simulink model "REV3"  (R2025b)
settings: Solver=ode8  StartTime=0.0  StopTime=inf  FixedStep=0.0001  RelTol=1e-3
undefined symbols (not defined in the file): BMS_Contactor_Command, MC_DC_State, MC_VSM_State, UC_State
(part 1 of 2)
settings Model: DataDictionary=rev3_data.sldd  PacingRate=0.001000  Creator=rebek  LastModifiedBy=diego
settings DebuggingCC: ParameterPrecisionLossMsg=none
settings RTWCC: GPUComputeCapability=3.5

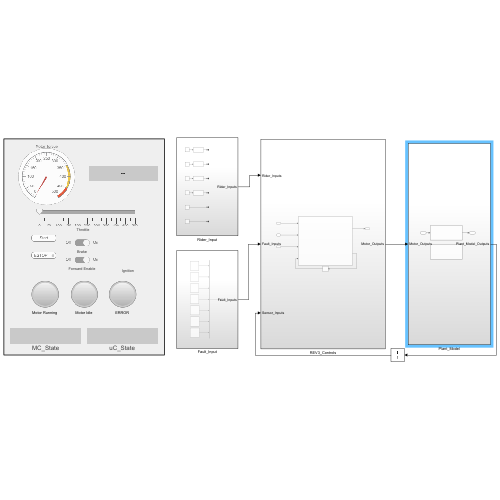
[thumbnail: Simulink's stored preview of the top-level diagram]
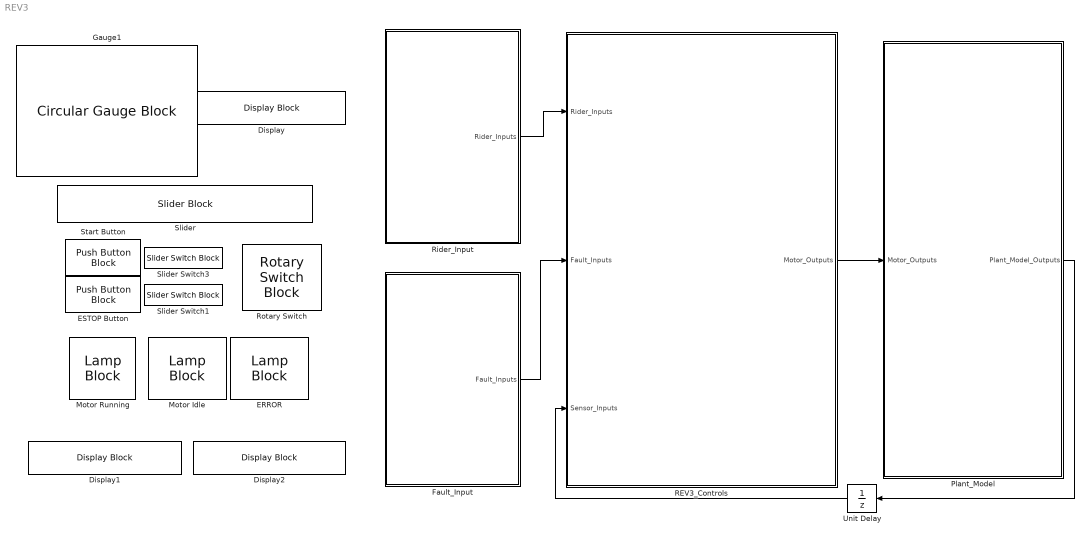
== system REV3 ==
  Display : DisplayBlock  LabelPosition=Hide  Transparency=1  GridColor=[0.502, 0.502, 0.502]
  Display1 : DisplayBlock  LabelPosition=Hide  Transparency=1  GridColor=[0.502, 0.502, 0.502]
      settings: AttributesFormatString=MC_State
  Display2 : DisplayBlock  LabelPosition=Hide  Transparency=1  GridColor=[0.502, 0.502, 0.502]
      settings: AttributesFormatString=uC_State
  ERROR : LampBlock  LabelPosition=Hide  DefaultColor=[192.0, 192.0, 192.0]
  ESTOP Button : PushButtonBlock  ButtonText=ESTOP  ButtonType=Latch  Icon=Circle  IconAlignment=Right  IconOnColor=[0.91764705882352937, 0.19607843137254902, 0.0392156862745098]  IconOffColor=[0.74901960784313726, 0.74901960784313726, 0.74901960784313726]  IconColor=On  OffValue=0.000000
  Fault_Input : Subsystem
  Gauge1 : CircularGaugeBlock  ScaleMax=500  FontColor=[0.0, 0.0, 0.0]
  Motor Idle : LampBlock  LabelPosition=Hide  DefaultColor=[192.0, 192.0, 192.0]
  Motor Running : LampBlock  LabelPosition=Hide  DefaultColor=[192.0, 192.0, 192.0]
  Plant_Model : Subsystem
  REV3_Controls : Subsystem
  Rider_Input : Subsystem
  Rotary Switch : RotarySwitchBlock  LabelPosition=Hide
      settings: AttributesFormatString=Ignition
  Slider : SliderBlock  LabelPosition=Hide  ScaleMax=500
      settings: AttributesFormatString=Throttle
  Slider Switch1 : SliderSwitchBlock  LabelPosition=Hide
      settings: AttributesFormatString=Forward Enable
  Slider Switch3 : SliderSwitchBlock  LabelPosition=Hide
      settings: AttributesFormatString=Brake
  Start Button : PushButtonBlock  ButtonText=Start  IconOnColor=[0.0, 0.39215686274509803, 0.0]  IconOffColor=[0.0, 1.0, 0.0]  OffValue=0.000000
  Unit Delay : UnitDelay  SampleTime=-1  HasFrameUpgradeWarning=on
  wires:
  Rider_Input/1(Rider_Inputs) -> REV3_Controls/1(Rider_Inputs)
  Fault_Input/1(Fault_Inputs) -> REV3_Controls/2(Fault_Inputs)
  REV3_Controls/1(Motor_Outputs) -> Plant_Model/1(Motor_Outputs)
  Plant_Model/1(Plant_Model_Outputs) -> Unit Delay/1
  Unit Delay/1 -> REV3_Controls/3(Sensor_Inputs)

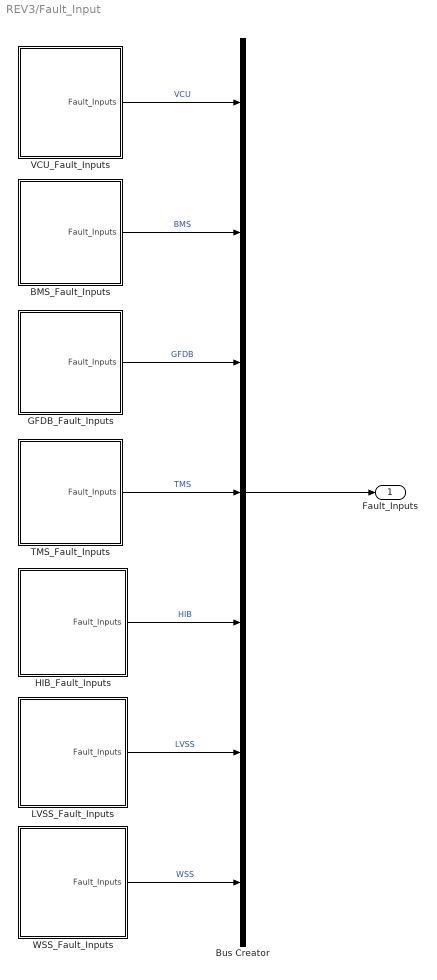
== system REV3/Fault_Input ==
  BMS_Fault_Inputs : Subsystem
  Bus Creator : BusCreator  Inputs=7
  GFDB_Fault_Inputs : Subsystem
  HIB_Fault_Inputs : Subsystem
  LVSS_Fault_Inputs : Subsystem
  TMS_Fault_Inputs : Subsystem
  VCU_Fault_Inputs : Subsystem
  WSS_Fault_Inputs : Subsystem
  Fault_Inputs : Outport
  wires:
  VCU_Fault_Inputs/1(Fault_Inputs) -> Bus Creator/1  "VCU"
  BMS_Fault_Inputs/1(Fault_Inputs) -> Bus Creator/2  "BMS"
  GFDB_Fault_Inputs/1(Fault_Inputs) -> Bus Creator/3  "GFDB"
  Bus Creator/1 -> Fault_Inputs/1
  TMS_Fault_Inputs/1(Fault_Inputs) -> Bus Creator/4  "TMS"
  HIB_Fault_Inputs/1(Fault_Inputs) -> Bus Creator/5  "HIB"
  LVSS_Fault_Inputs/1(Fault_Inputs) -> Bus Creator/6  "LVSS"
  WSS_Fault_Inputs/1(Fault_Inputs) -> Bus Creator/7  "WSS"

== system REV3/Plant_Model ==
  Motor_Outputs : Inport
  Bike_Orientation : Subsystem
  Wheel_Speed : Subsystem
  Plant_Model_Outputs : Outport
  wires:
  Motor_Outputs/1 -> Wheel_Speed/1(Motor_Outputs)
  Wheel_Speed/1(Plant_Model_Outputs) -> Plant_Model_Outputs/1

== system REV3/REV3_Controls ==
  Rider_Inputs : Inport
  Fault_Inputs : Inport  Port=2
  Sensor_Inputs : Inport  Port=3
  Control_Step : Subsystem
  Unit Delay : UnitDelay  SampleTime=-1  HasFrameUpgradeWarning=on
  Motor_Outputs : Outport
  wires:
  Rider_Inputs/1 -> Control_Step/1(Rider_Inputs)
  Fault_Inputs/1 -> Control_Step/2(Fault_Inputs)
  Unit Delay/1 -> Control_Step/4(Feedback_Input)
  Control_Step/1(Motor_Outputs) -> Motor_Outputs/1
  Control_Step/2(Feedback_Output) -> Unit Delay/1
  Sensor_Inputs/1 -> Control_Step/3(Sensor_Inputs)

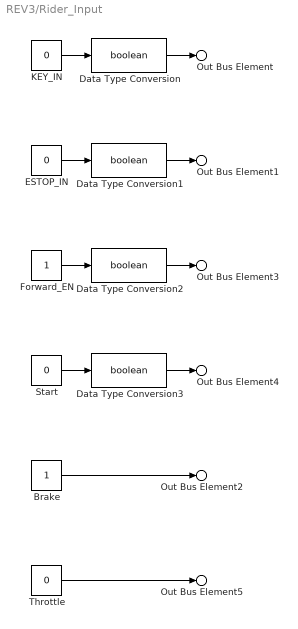
== system REV3/Rider_Input ==
  Brake : Constant
  Data Type Conversion{,1..3} (4 alike) : DataTypeConversion  OutDataTypeStr=boolean  SaturateOnIntegerOverflow=off  RndMeth=Floor
  ESTOP_IN : Constant  Value=0
  Forward_EN : Constant
  KEY_IN : Constant  Value=0
  Start : Constant  Value=0
  Throttle : Constant  Value=0  OutDataTypeStr=int16
  Out Bus Element5 : Outport  PortName=Rider_Inputs  Element=Yes_HIB.Throttle
  Out Bus Element4 : Outport  PortName=Rider_Inputs  Element=Yes_HIB.Start
  Out Bus Element3 : Outport  PortName=Rider_Inputs  Element=Yes_HIB.Forward_EN
  Out Bus Element2 : Outport  PortName=Rider_Inputs  Element=Yes_HIB.Brake
  Out Bus Element : Outport  PortName=Rider_Inputs  Element=No_HIB.Key_In
  Out Bus Element1 : Outport  PortName=Rider_Inputs  Element=No_HIB.Estop_In
  wires:
  KEY_IN/1 -> Data Type Conversion/1
  Brake/1 -> Out Bus Element2/1
  Data Type Conversion2/1 -> Out Bus Element3/1
  Data Type Conversion/1 -> Out Bus Element/1
  Forward_EN/1 -> Data Type Conversion2/1
  Data Type Conversion3/1 -> Out Bus Element4/1
  ESTOP_IN/1 -> Data Type Conversion1/1
  Throttle/1 -> Out Bus Element5/1
  Data Type Conversion1/1 -> Out Bus Element1/1
  Start/1 -> Data Type Conversion3/1

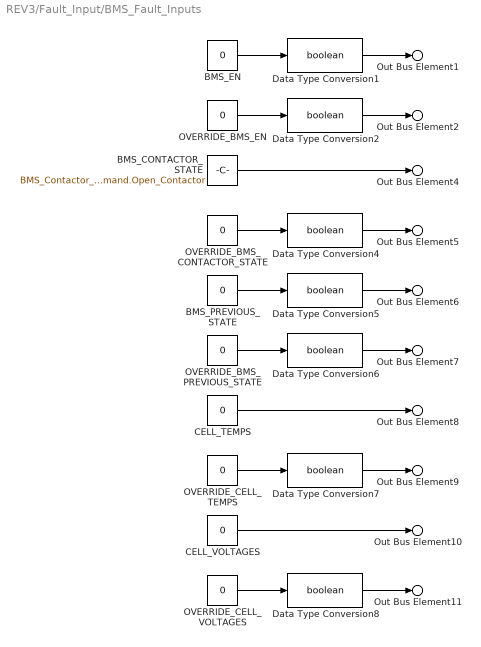
== system REV3/Fault_Input/BMS_Fault_Inputs ==
  BMS_CONTACTOR_STATE : Constant  Value=BMS_Contactor_Command.Open_Contactor  OutDataTypeStr=Enum: BMS_Contactor_Command
  BMS_EN : Constant  Value=0
  BMS_PREVIOUS_STATE : Constant  Value=0
  CELL_TEMPS : Constant  Value=0
  CELL_VOLTAGES : Constant  Value=0
  Data Type Conversion{1..2,4..8} (7 alike) : DataTypeConversion  OutDataTypeStr=boolean  SaturateOnIntegerOverflow=off  RndMeth=Floor
  OVERRIDE_BMS_CONTACTOR_STATE : Constant  Value=0
  OVERRIDE_BMS_EN : Constant  Value=0
  OVERRIDE_BMS_PREVIOUS_STATE : Constant  Value=0
  OVERRIDE_CELL_TEMPS : Constant  Value=0
  OVERRIDE_CELL_VOLTAGES : Constant  Value=0
  Out Bus Element4 : Outport  PortName=Fault_Inputs  Element=BMS_Contactor_State
  Out Bus Element5 : Outport  PortName=Fault_Inputs  Element=Override_BMS_Contactor_State
  Out Bus Element6 : Outport  PortName=Fault_Inputs  Element=BMS_Previous_State
  Out Bus Element7 : Outport  PortName=Fault_Inputs  Element=Override_BMS_Previous_State
  Out Bus Element8 : Outport  PortName=Fault_Inputs  Element=Cell_Temps
  Out Bus Element9 : Outport  PortName=Fault_Inputs  Element=Override_Cell_Temps
  Out Bus Element10 : Outport  PortName=Fault_Inputs  Element=Cell_Voltages
  Out Bus Element11 : Outport  PortName=Fault_Inputs  Element=Override_Cell_Voltages
  Out Bus Element1 : Outport  PortName=Fault_Inputs  Element=BMS_EN
  Out Bus Element2 : Outport  PortName=Fault_Inputs  Element=Override_BMS_EN
  wires:
  CELL_VOLTAGES/1 -> Out Bus Element10/1
  Data Type Conversion7/1 -> Out Bus Element9/1
  BMS_PREVIOUS_STATE/1 -> Data Type Conversion5/1
  OVERRIDE_CELL_TEMPS/1 -> Data Type Conversion7/1
  OVERRIDE_BMS_PREVIOUS_STATE/1 -> Data Type Conversion6/1
  BMS_CONTACTOR_STATE/1 -> Out Bus Element4/1
  OVERRIDE_CELL_VOLTAGES/1 -> Data Type Conversion8/1
  Data Type Conversion4/1 -> Out Bus Element5/1
  OVERRIDE_BMS_CONTACTOR_STATE/1 -> Data Type Conversion4/1
  Data Type Conversion5/1 -> Out Bus Element6/1
  Data Type Conversion6/1 -> Out Bus Element7/1
  CELL_TEMPS/1 -> Out Bus Element8/1
  Data Type Conversion8/1 -> Out Bus Element11/1
  Data Type Conversion2/1 -> Out Bus Element2/1
  Data Type Conversion1/1 -> Out Bus Element1/1
  BMS_EN/1 -> Data Type Conversion1/1
  OVERRIDE_BMS_EN/1 -> Data Type Conversion2/1

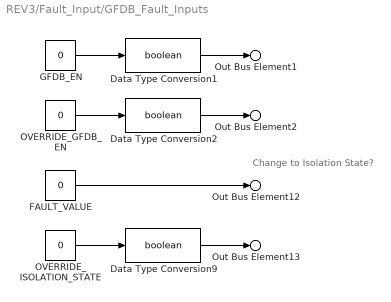
== system REV3/Fault_Input/GFDB_Fault_Inputs ==
  note: Change to Isolation State?
  Data Type Conversion1 : DataTypeConversion  OutDataTypeStr=boolean  SaturateOnIntegerOverflow=off  RndMeth=Floor
  Data Type Conversion2 : DataTypeConversion  OutDataTypeStr=boolean  SaturateOnIntegerOverflow=off  RndMeth=Floor
  Data Type Conversion9 : DataTypeConversion  OutDataTypeStr=boolean  SaturateOnIntegerOverflow=off  RndMeth=Floor
  FAULT_VALUE : Constant  Value=0
  GFDB_EN : Constant  Value=0
  OVERRIDE_GFDB_EN : Constant  Value=0
  OVERRIDE_ISOLATION_STATE : Constant  Value=0
  Out Bus Element12 : Outport  PortName=Fault_Inputs  Element=Fault_Value
  Out Bus Element13 : Outport  PortName=Fault_Inputs  Element=Override_Isolation_State
  Out Bus Element1 : Outport  PortName=Fault_Inputs  Element=GFDB_EN
  Out Bus Element2 : Outport  PortName=Fault_Inputs  Element=Override_GFDB_EN
  wires:
  FAULT_VALUE/1 -> Out Bus Element12/1
  Data Type Conversion9/1 -> Out Bus Element13/1
  OVERRIDE_ISOLATION_STATE/1 -> Data Type Conversion9/1
  OVERRIDE_GFDB_EN/1 -> Data Type Conversion2/1
  Data Type Conversion2/1 -> Out Bus Element2/1
  Data Type Conversion1/1 -> Out Bus Element1/1
  GFDB_EN/1 -> Data Type Conversion1/1

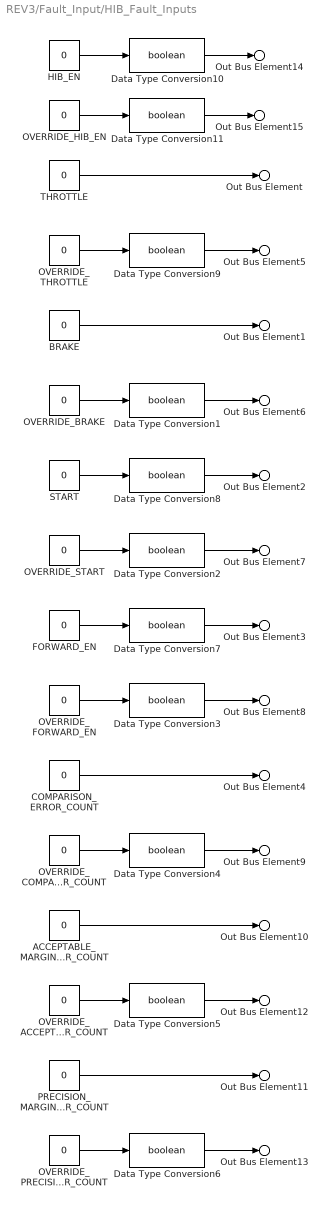
== system REV3/Fault_Input/HIB_Fault_Inputs ==
  ACCEPTABLE_MARGIN_ERROR_COUNT : Constant  Value=0
  BRAKE : Constant  Value=0
  COMPARISON_ERROR_COUNT : Constant  Value=0
  Data Type Conversion{1..11} (11 alike) : DataTypeConversion  OutDataTypeStr=boolean  SaturateOnIntegerOverflow=off  RndMeth=Floor
  FORWARD_EN : Constant  Value=0
  HIB_EN : Constant  Value=0
  OVERRIDE_ACCEPTABLE_MARGIN_ERROR_COUNT : Constant  Value=0
  OVERRIDE_BRAKE : Constant  Value=0
  OVERRIDE_COMPARISON_ERROR_COUNT : Constant  Value=0
  OVERRIDE_FORWARD_EN : Constant  Value=0
  OVERRIDE_HIB_EN : Constant  Value=0
  OVERRIDE_PRECISION_MARGIN_ERROR_COUNT : Constant  Value=0
  OVERRIDE_START : Constant  Value=0
  OVERRIDE_THROTTLE : Constant  Value=0
  PRECISION_MARGIN_ERROR_COUNT : Constant  Value=0
  START : Constant  Value=0
  THROTTLE : Constant  Value=0
  Out Bus Element : Outport  PortName=Fault_Inputs  Element=Throttle
  Out Bus Element1 : Outport  PortName=Fault_Inputs  Element=Brake
  Out Bus Element2 : Outport  PortName=Fault_Inputs  Element=Start
  Out Bus Element3 : Outport  PortName=Fault_Inputs  Element=Forward_EN
  Out Bus Element4 : Outport  PortName=Fault_Inputs  Element=Comparison_Error_Count
  Out Bus Element5 : Outport  PortName=Fault_Inputs  Element=Override_Throttle
  Out Bus Element6 : Outport  PortName=Fault_Inputs  Element=Override_Brake
  Out Bus Element7 : Outport  PortName=Fault_Inputs  Element=Override_Start
  Out Bus Element8 : Outport  PortName=Fault_Inputs  Element=Override_Forward_EN
  Out Bus Element9 : Outport  PortName=Fault_Inputs  Element=Override_Comparison_Error_Count
  Out Bus Element10 : Outport  PortName=Fault_Inputs  Element=Acceptable_Margin_Error_Count
  Out Bus Element11 : Outport  PortName=Fault_Inputs  Element=Precision_Margin_Error_Count
  Out Bus Element12 : Outport  PortName=Fault_Inputs  Element=Override_Acceptable_Margin_Error_Count
  Out Bus Element13 : Outport  PortName=Fault_Inputs  Element=Override_Precision_Margin_Error_Count
  Out Bus Element14 : Outport  PortName=Fault_Inputs  Element=HIB_EN
  Out Bus Element15 : Outport  PortName=Fault_Inputs  Element=Override_HIB_EN
  wires:
  THROTTLE/1 -> Out Bus Element/1
  BRAKE/1 -> Out Bus Element1/1
  FORWARD_EN/1 -> Data Type Conversion7/1
  START/1 -> Data Type Conversion8/1
  COMPARISON_ERROR_COUNT/1 -> Out Bus Element4/1
  OVERRIDE_THROTTLE/1 -> Data Type Conversion9/1
  Data Type Conversion9/1 -> Out Bus Element5/1
  Data Type Conversion1/1 -> Out Bus Element6/1
  OVERRIDE_BRAKE/1 -> Data Type Conversion1/1
  Data Type Conversion2/1 -> Out Bus Element7/1
  OVERRIDE_START/1 -> Data Type Conversion2/1
  Data Type Conversion3/1 -> Out Bus Element8/1
  OVERRIDE_FORWARD_EN/1 -> Data Type Conversion3/1
  Data Type Conversion4/1 -> Out Bus Element9/1
  OVERRIDE_COMPARISON_ERROR_COUNT/1 -> Data Type Conversion4/1
  PRECISION_MARGIN_ERROR_COUNT/1 -> Out Bus Element11/1
  Data Type Conversion6/1 -> Out Bus Element13/1
  Data Type Conversion5/1 -> Out Bus Element12/1
  ACCEPTABLE_MARGIN_ERROR_COUNT/1 -> Out Bus Element10/1
  OVERRIDE_ACCEPTABLE_MARGIN_ERROR_COUNT/1 -> Data Type Conversion5/1
  OVERRIDE_PRECISION_MARGIN_ERROR_COUNT/1 -> Data Type Conversion6/1
  Data Type Conversion7/1 -> Out Bus Element3/1
  Data Type Conversion8/1 -> Out Bus Element2/1
  OVERRIDE_HIB_EN/1 -> Data Type Conversion11/1
  Data Type Conversion11/1 -> Out Bus Element15/1
  Data Type Conversion10/1 -> Out Bus Element14/1
  HIB_EN/1 -> Data Type Conversion10/1

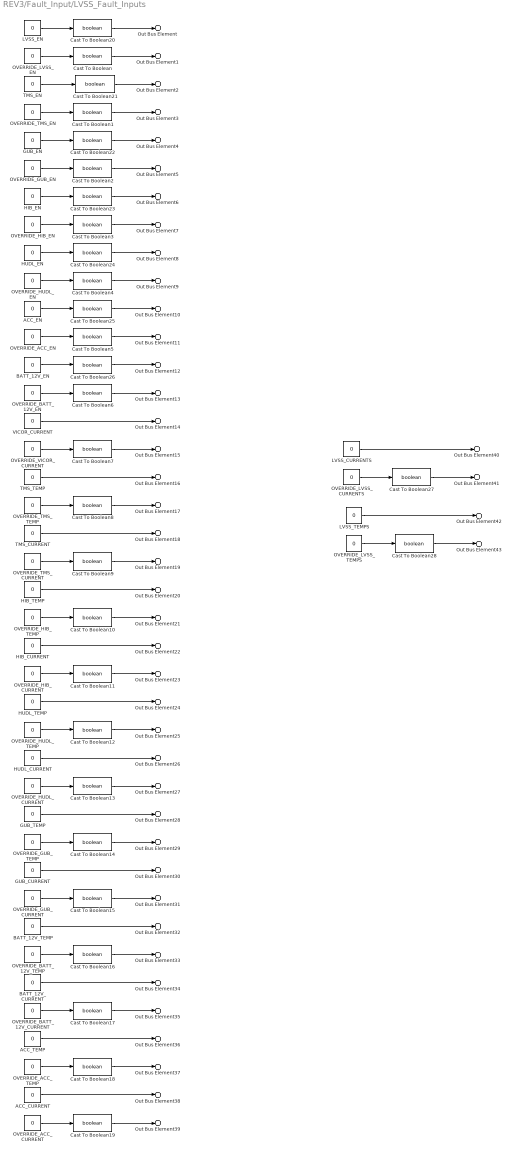
== system REV3/Fault_Input/LVSS_Fault_Inputs ==
  ACC_CURRENT : Constant  Value=0
  ACC_EN : Constant  Value=0
  ACC_TEMP : Constant  Value=0
  BATT_12V_CURRENT : Constant  Value=0
  BATT_12V_EN : Constant  Value=0
  BATT_12V_TEMP : Constant  Value=0
  Cast To Boolean{,1..28} (29 alike) : DataTypeConversion  OutDataTypeStr=boolean  SaturateOnIntegerOverflow=off  RndMeth=Floor
  GUB_CURRENT : Constant  Value=0
  GUB_EN : Constant  Value=0
  GUB_TEMP : Constant  Value=0
  HIB_CURRENT : Constant  Value=0
  HIB_EN : Constant  Value=0
  HIB_TEMP : Constant  Value=0
  HUDL_CURRENT : Constant  Value=0
  HUDL_EN : Constant  Value=0
  HUDL_TEMP : Constant  Value=0
  LVSS_CURRENTS : Constant  Value=0
  LVSS_EN : Constant  Value=0
  LVSS_TEMPS : Constant  Value=0
  OVERRIDE_ACC_CURRENT : Constant  Value=0
  OVERRIDE_ACC_EN : Constant  Value=0
  OVERRIDE_ACC_TEMP : Constant  Value=0
  OVERRIDE_BATT_12V_CURRENT : Constant  Value=0
  OVERRIDE_BATT_12V_EN : Constant  Value=0
  OVERRIDE_BATT_12V_TEMP : Constant  Value=0
  OVERRIDE_GUB_CURRENT : Constant  Value=0
  OVERRIDE_GUB_EN : Constant  Value=0
  OVERRIDE_GUB_TEMP : Constant  Value=0
  OVERRIDE_HIB_CURRENT : Constant  Value=0
  OVERRIDE_HIB_EN : Constant  Value=0
  OVERRIDE_HIB_TEMP : Constant  Value=0
  OVERRIDE_HUDL_CURRENT : Constant  Value=0
  OVERRIDE_HUDL_EN : Constant  Value=0
  OVERRIDE_HUDL_TEMP : Constant  Value=0
  OVERRIDE_LVSS_CURRENTS : Constant  Value=0
  OVERRIDE_LVSS_EN : Constant  Value=0
  OVERRIDE_LVSS_TEMPS : Constant  Value=0
  OVERRIDE_TMS_CURRENT : Constant  Value=0
  OVERRIDE_TMS_EN : Constant  Value=0
  OVERRIDE_TMS_TEMP : Constant  Value=0
  OVERRIDE_VICOR_CURRENT : Constant  Value=0
  TMS_CURRENT : Constant  Value=0
  TMS_EN : Constant  Value=0
  TMS_TEMP : Constant  Value=0
  VICOR_CURRENT : Constant  Value=0
  Out Bus Element : Outport  PortName=Fault_Inputs  Element=LVSS_EN
  Out Bus Element1 : Outport  PortName=Fault_Inputs  Element=Override_LVSS_EN
  Out Bus Element2 : Outport  PortName=Fault_Inputs  Element=TMS_EN
  Out Bus Element3 : Outport  PortName=Fault_Inputs  Element=Override_TMS_EN
  Out Bus Element4 : Outport  PortName=Fault_Inputs  Element=GUB_EN
  Out Bus Element5 : Outport  PortName=Fault_Inputs  Element=Override_GUB_EN
  Out Bus Element6 : Outport  PortName=Fault_Inputs  Element=HIB_EN
  Out Bus Element7 : Outport  PortName=Fault_Inputs  Element=Override_HIB_EN
  Out Bus Element8 : Outport  PortName=Fault_Inputs  Element=HUDL_EN
  Out Bus Element9 : Outport  PortName=Fault_Inputs  Element=Override_HUDL_EN
  Out Bus Element10 : Outport  PortName=Fault_Inputs  Element=Acc_EN
  Out Bus Element11 : Outport  PortName=Fault_Inputs  Element=Override_Acc_EN
  Out Bus Element12 : Outport  PortName=Fault_Inputs  Element=Batt_12V_EN
  Out Bus Element13 : Outport  PortName=Fault_Inputs  Element=Override_Batt_12V_EN
  Out Bus Element14 : Outport  PortName=Fault_Inputs  Element=Vicor_Current
  Out Bus Element15 : Outport  PortName=Fault_Inputs  Element=Override_Vicor_Current
  Out Bus Element16 : Outport  PortName=Fault_Inputs  Element=TMS_Temp
  Out Bus Element17 : Outport  PortName=Fault_Inputs  Element=Override_TMS_Temp
  Out Bus Element18 : Outport  PortName=Fault_Inputs  Element=TMS_Current
  Out Bus Element19 : Outport  PortName=Fault_Inputs  Element=Override_TMS_Current
  Out Bus Element20 : Outport  PortName=Fault_Inputs  Element=HIB_Temp
  Out Bus Element21 : Outport  PortName=Fault_Inputs  Element=Override_HIB_Temp
  Out Bus Element22 : Outport  PortName=Fault_Inputs  Element=HIB_Current
  Out Bus Element23 : Outport  PortName=Fault_Inputs  Element=Override_HIB_Current
  Out Bus Element24 : Outport  PortName=Fault_Inputs  Element=HUDL_Temp
  Out Bus Element25 : Outport  PortName=Fault_Inputs  Element=Override_HUDL_Temp
  Out Bus Element26 : Outport  PortName=Fault_Inputs  Element=HUDL_Current
  Out Bus Element27 : Outport  PortName=Fault_Inputs  Element=Override_HUDL_Current
  Out Bus Element28 : Outport  PortName=Fault_Inputs  Element=GUB_Temp
  Out Bus Element29 : Outport  PortName=Fault_Inputs  Element=Override_GUB_Temp
  Out Bus Element30 : Outport  PortName=Fault_Inputs  Element=GUB_Current
  Out Bus Element31 : Outport  PortName=Fault_Inputs  Element=Override_GUB_Current
  Out Bus Element32 : Outport  PortName=Fault_Inputs  Element=Batt_12V_Temp
  Out Bus Element33 : Outport  PortName=Fault_Inputs  Element=Override_Batt_12V_Temp
  Out Bus Element34 : Outport  PortName=Fault_Inputs  Element=Batt_12V_Current
  Out Bus Element35 : Outport  PortName=Fault_Inputs  Element=Override_Batt_12V_Current
  Out Bus Element36 : Outport  PortName=Fault_Inputs  Element=Acc_Temp
  Out Bus Element37 : Outport  PortName=Fault_Inputs  Element=Override_Acc_Temp
  Out Bus Element38 : Outport  PortName=Fault_Inputs  Element=Acc_Current
  Out Bus Element39 : Outport  PortName=Fault_Inputs  Element=Override_Acc_Current
  Out Bus Element40 : Outport  PortName=Fault_Inputs  Element=LVSS_Currents
  Out Bus Element41 : Outport  PortName=Fault_Inputs  Element=Override_LVSS_Currents
  Out Bus Element42 : Outport  PortName=Fault_Inputs  Element=LVSS_Temps
  Out Bus Element43 : Outport  PortName=Fault_Inputs  Element=Override_LVSS_Temps
  wires:
  OVERRIDE_ACC_CURRENT/1 -> Cast To Boolean19/1
  OVERRIDE_ACC_TEMP/1 -> Cast To Boolean18/1
  OVERRIDE_BATT_12V_CURRENT/1 -> Cast To Boolean17/1
  OVERRIDE_BATT_12V_TEMP/1 -> Cast To Boolean16/1
  OVERRIDE_GUB_CURRENT/1 -> Cast To Boolean15/1
  OVERRIDE_GUB_TEMP/1 -> Cast To Boolean14/1
  OVERRIDE_HUDL_CURRENT/1 -> Cast To Boolean13/1
  OVERRIDE_HUDL_TEMP/1 -> Cast To Boolean12/1
  OVERRIDE_HIB_CURRENT/1 -> Cast To Boolean11/1
  OVERRIDE_HIB_TEMP/1 -> Cast To Boolean10/1
  OVERRIDE_TMS_CURRENT/1 -> Cast To Boolean9/1
  OVERRIDE_TMS_TEMP/1 -> Cast To Boolean8/1
  OVERRIDE_VICOR_CURRENT/1 -> Cast To Boolean7/1
  OVERRIDE_BATT_12V_EN/1 -> Cast To Boolean6/1
  OVERRIDE_ACC_EN/1 -> Cast To Boolean5/1
  OVERRIDE_HUDL_EN/1 -> Cast To Boolean4/1
  OVERRIDE_HIB_EN/1 -> Cast To Boolean3/1
  OVERRIDE_GUB_EN/1 -> Cast To Boolean2/1
  OVERRIDE_TMS_EN/1 -> Cast To Boolean1/1
  OVERRIDE_LVSS_EN/1 -> Cast To Boolean/1
  Cast To Boolean19/1 -> Out Bus Element39/1
  ACC_CURRENT/1 -> Out Bus Element38/1
  Cast To Boolean18/1 -> Out Bus Element37/1
  ACC_TEMP/1 -> Out Bus Element36/1
  Cast To Boolean17/1 -> Out Bus Element35/1
  BATT_12V_CURRENT/1 -> Out Bus Element34/1
  Cast To Boolean16/1 -> Out Bus Element33/1
  BATT_12V_TEMP/1 -> Out Bus Element32/1
  Cast To Boolean15/1 -> Out Bus Element31/1
  GUB_CURRENT/1 -> Out Bus Element30/1
  Cast To Boolean14/1 -> Out Bus Element29/1
  GUB_TEMP/1 -> Out Bus Element28/1
  Cast To Boolean13/1 -> Out Bus Element27/1
  HUDL_CURRENT/1 -> Out Bus Element26/1
  Cast To Boolean12/1 -> Out Bus Element25/1
  HUDL_TEMP/1 -> Out Bus Element24/1
  Cast To Boolean11/1 -> Out Bus Element23/1
  HIB_CURRENT/1 -> Out Bus Element22/1
  Cast To Boolean10/1 -> Out Bus Element21/1
  HIB_TEMP/1 -> Out Bus Element20/1
  Cast To Boolean9/1 -> Out Bus Element19/1
  TMS_CURRENT/1 -> Out Bus Element18/1
  Cast To Boolean8/1 -> Out Bus Element17/1
  TMS_TEMP/1 -> Out Bus Element16/1
  Cast To Boolean7/1 -> Out Bus Element15/1
  Cast To Boolean6/1 -> Out Bus Element13/1
  BATT_12V_EN/1 -> Cast To Boolean26/1
  Cast To Boolean5/1 -> Out Bus Element11/1
  ACC_EN/1 -> Cast To Boolean25/1
  Cast To Boolean4/1 -> Out Bus Element9/1
  HUDL_EN/1 -> Cast To Boolean24/1
  Cast To Boolean3/1 -> Out Bus Element7/1
  HIB_EN/1 -> Cast To Boolean23/1
  Cast To Boolean2/1 -> Out Bus Element5/1
  GUB_EN/1 -> Cast To Boolean22/1
  Cast To Boolean1/1 -> Out Bus Element3/1
  TMS_EN/1 -> Cast To Boolean21/1
  Cast To Boolean/1 -> Out Bus Element1/1
  LVSS_EN/1 -> Cast To Boolean20/1
  Cast To Boolean20/1 -> Out Bus Element/1
  Cast To Boolean21/1 -> Out Bus Element2/1
  Cast To Boolean22/1 -> Out Bus Element4/1
  Cast To Boolean23/1 -> Out Bus Element6/1
  Cast To Boolean24/1 -> Out Bus Element8/1
  Cast To Boolean25/1 -> Out Bus Element10/1
  Cast To Boolean26/1 -> Out Bus Element12/1
  VICOR_CURRENT/1 -> Out Bus Element14/1
  Cast To Boolean27/1 -> Out Bus Element41/1
  OVERRIDE_LVSS_CURRENTS/1 -> Cast To Boolean27/1
  LVSS_CURRENTS/1 -> Out Bus Element40/1
  Cast To Boolean28/1 -> Out Bus Element43/1
  OVERRIDE_LVSS_TEMPS/1 -> Cast To Boolean28/1
  LVSS_TEMPS/1 -> Out Bus Element42/1

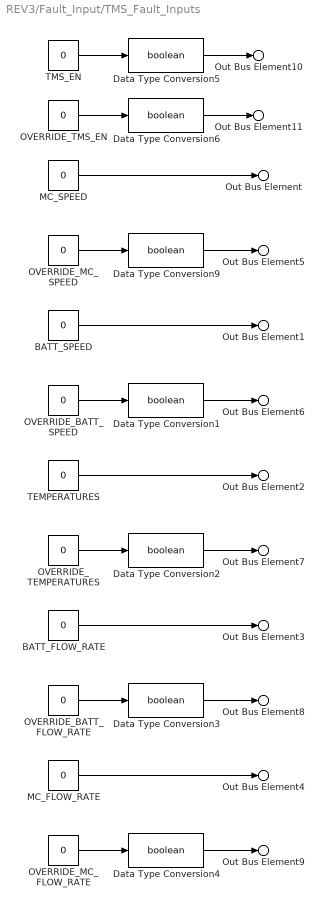
== system REV3/Fault_Input/TMS_Fault_Inputs ==
  BATT_FLOW_RATE : Constant  Value=0
  BATT_SPEED : Constant  Value=0
  Data Type Conversion{1..6,9} (7 alike) : DataTypeConversion  OutDataTypeStr=boolean  SaturateOnIntegerOverflow=off  RndMeth=Floor
  MC_FLOW_RATE : Constant  Value=0
  MC_SPEED : Constant  Value=0
  OVERRIDE_BATT_FLOW_RATE : Constant  Value=0
  OVERRIDE_BATT_SPEED : Constant  Value=0
  OVERRIDE_MC_FLOW_RATE : Constant  Value=0
  OVERRIDE_MC_SPEED : Constant  Value=0
  OVERRIDE_TEMPERATURES : Constant  Value=0
  OVERRIDE_TMS_EN : Constant  Value=0
  TEMPERATURES : Constant  Value=0
  TMS_EN : Constant  Value=0
  Out Bus Element : Outport  PortName=Fault_Inputs  Element=MC_Speed
  Out Bus Element1 : Outport  PortName=Fault_Inputs  Element=Batt_Speed
  Out Bus Element2 : Outport  PortName=Fault_Inputs  Element=Temperatures
  Out Bus Element3 : Outport  PortName=Fault_Inputs  Element=Batt_Flow_Rate
  Out Bus Element4 : Outport  PortName=Fault_Inputs  Element=MC_Flow_Rate
  Out Bus Element5 : Outport  PortName=Fault_Inputs  Element=Override_MC_Speed
  Out Bus Element6 : Outport  PortName=Fault_Inputs  Element=Override_Batt_Speed
  Out Bus Element7 : Outport  PortName=Fault_Inputs  Element=Override_Temperatures
  Out Bus Element8 : Outport  PortName=Fault_Inputs  Element=Override_Batt_FR
  Out Bus Element9 : Outport  PortName=Fault_Inputs  Element=Override_MC_FR
  Out Bus Element10 : Outport  PortName=Fault_Inputs  Element=TMS_EN
  Out Bus Element11 : Outport  PortName=Fault_Inputs  Element=Override_TMS_EN
  wires:
  MC_SPEED/1 -> Out Bus Element/1
  BATT_SPEED/1 -> Out Bus Element1/1
  BATT_FLOW_RATE/1 -> Out Bus Element3/1
  TEMPERATURES/1 -> Out Bus Element2/1
  MC_FLOW_RATE/1 -> Out Bus Element4/1
  OVERRIDE_MC_SPEED/1 -> Data Type Conversion9/1
  Data Type Conversion9/1 -> Out Bus Element5/1
  Data Type Conversion1/1 -> Out Bus Element6/1
  OVERRIDE_BATT_SPEED/1 -> Data Type Conversion1/1
  Data Type Conversion2/1 -> Out Bus Element7/1
  OVERRIDE_TEMPERATURES/1 -> Data Type Conversion2/1
  Data Type Conversion3/1 -> Out Bus Element8/1
  OVERRIDE_BATT_FLOW_RATE/1 -> Data Type Conversion3/1
  Data Type Conversion4/1 -> Out Bus Element9/1
  OVERRIDE_MC_FLOW_RATE/1 -> Data Type Conversion4/1
  OVERRIDE_TMS_EN/1 -> Data Type Conversion6/1
  Data Type Conversion6/1 -> Out Bus Element11/1
  Data Type Conversion5/1 -> Out Bus Element10/1
  TMS_EN/1 -> Data Type Conversion5/1

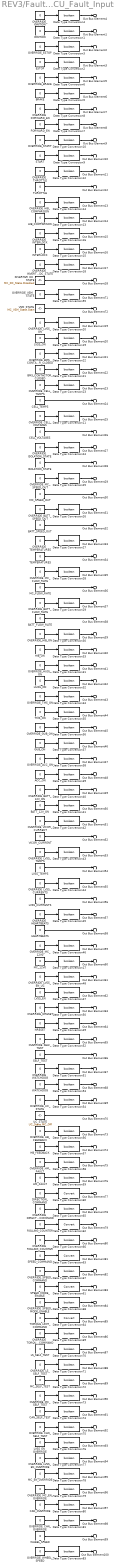
== system REV3/Fault_Input/VCU_Fault_Inputs ==
  ACC_ON : Constant  Value=0
  BATT_12V_ON : Constant  Value=0
  BATT_FLOW_RATE : Constant  Value=0
  BATT_SPEED_OUT : Constant  Value=0
  BMS_CONTACTOR_CLOSED : Constant  Value=0
  BRAKE : Constant  Value=0
  CAN_OVERRIDE : Constant  Value=0
  CAN_SELF_TEST : Constant  Value=0
  CELL_TEMPS : Constant  Value=0
  CELL_VOLTAGES : Constant  Value=0
  DIRECTION_COMMAND : Constant  Value=0
  Data Type Conversion{1..59,65..81,83} (77 alike) : DataTypeConversion  OutDataTypeStr=boolean  SaturateOnIntegerOverflow=off  RndMeth=Floor
  Data Type Conversion{60..64} (5 alike) : DataTypeConversion  SaturateOnIntegerOverflow=off  RndMeth=Floor
  ESTOP : Constant  Value=0
  FORWARD_EN : Constant  Value=0
  GUB_ON : Constant  Value=0
  HB_FEEDBACK : Constant  Value=0
  HEARTBEATS : Constant  Value=0
  HIB_COMPARISON : Constant  Value=0
  HIB_ON : Constant  Value=0
  HM_FAULT : Constant  Value=0
  HUDL_ON : Constant  Value=0
  IGNITION : Constant  Value=0
  INTERLOCK : Constant  Value=0
  INVERTER_DC_STATE : Constant  Value=MC_DC_State.Disabled
  ISOLATION_STATE : Constant  Value=0
  LS_SELF_TEST : Constant  Value=0
  LVSS_CURRENTS : Constant  Value=0
  LVSS_EN : Constant  Value=0
  LVSS_EN_OVERRIDE : Constant  Value=0
  LVSS_ON : Constant  Value=0
  LVSS_TEMPS : Constant  Value=0
  MC_12V0 : Constant  Value=0
  MC_EN_OVERRIDE : Constant  Value=0
  MC_FLOW_RATE : Constant  Value=0
  MC_SELF_TEST : Constant  Value=0
  MC_SPEED_OUT : Constant  Value=0
  NRESET : Constant  Value=0
  OVERRIDE_ACC_ON : Constant  Value=0
  OVERRIDE_BATT_12V_ON : Constant  Value=0
  OVERRIDE_BATT_FLOW_RATE : Constant  Value=0
  OVERRIDE_BATT_SPEED_OUT : Constant  Value=0
  OVERRIDE_BMS_CONTACTOR_CLOSED : Constant  Value=0
  OVERRIDE_BRAKE : Constant  Value=0
  OVERRIDE_CAN_OVERRIDE : Constant  Value=0
  OVERRIDE_CAN_SELF_TEST : Constant  Value=0
  OVERRIDE_CELL_TEMPS : Constant  Value=0
  OVERRIDE_CELL_VOLTAGES : Constant  Value=0
  OVERRIDE_DIRECTION_COMMAND : Constant  Value=0
  OVERRIDE_ESTOP : Constant  Value=0
  OVERRIDE_FORWARD_EN : Constant  Value=0
  OVERRIDE_GUB_ON : Constant  Value=0
  OVERRIDE_HB_FEEDBACK : Constant  Value=0
  OVERRIDE_HEARTBEATS : Constant  Value=0
  OVERRIDE_HIB_COMPARISON : Constant  Value=0
  OVERRIDE_HIB_ON : Constant  Value=0
  OVERRIDE_HM_FAULT : Constant  Value=0
  OVERRIDE_HUDL_ON : Constant  Value=0
  OVERRIDE_IGNITION : Constant  Value=0
  OVERRIDE_INTERLOCK : Constant  Value=0
  OVERRIDE_INVERTER_DC_STATE : Constant  Value=0
  OVERRIDE_ISOLATION_STATE : Constant  Value=0
  OVERRIDE_LS_SELF_TEST : Constant  Value=0
  OVERRIDE_LVSS_CURRENTS : Constant  Value=0
  OVERRIDE_LVSS_EN_OVERRIDE : Constant  Value=0
  OVERRIDE_LVSS_EN_UC : Constant  Value=0
  OVERRIDE_LVSS_ON : Constant  Value=0
  OVERRIDE_LVSS_TEMPS : Constant  Value=0
  OVERRIDE_MC_12V0 : Constant  Value=0
  OVERRIDE_MC_EN_OVERRIDE : Constant  Value=0
  OVERRIDE_MC_FLOW_RATE : Constant  Value=0
  OVERRIDE_MC_SELF_TEST : Constant  Value=0
  OVERRIDE_MC_SPEED_OUT : Constant  Value=0
  OVERRIDE_NRESET : Constant  Value=0
  OVERRIDE_ROLLING_COUNTER : Constant  Value=0
  OVERRIDE_SELF_TEST : Constant  Value=0
  OVERRIDE_SPEED_COMMAND : Constant  Value=0
  OVERRIDE_SPEED_MODE_ENABLE : Constant  Value=0
  OVERRIDE_START : Constant  Value=0
  OVERRIDE_TEMPERATURES : Constant  Value=0
  OVERRIDE_THROTTLE : Constant  Value=0
  OVERRIDE_TMS_ON : Constant  Value=0
  OVERRIDE_TORQUE_LIMIT_COMMAND : Constant  Value=0
  OVERRIDE_UC_STATE : Constant  Value=0
  OVERRIDE_VICOR_CURRENT : Constant  Value=0
  OVERRIDE_VSM_STATE : Constant  Value=0
  OVERRIDE_WATCHDOG : Constant  Value=0
  OVERRIDE_WHEEL_SPEED : Constant  Value=0
  ROLLING_COUNTER : Constant  Value=0
  SELF_TEST : Constant  Value=0
  SPEED_COMMAND : Constant  Value=0
  SPEED_MODE_ENABLE : Constant  Value=0
  START : Constant  Value=0
  TEMPERATURES : Constant  Value=0
  THROTTLE : Constant  Value=0
  TMS_ON : Constant  Value=0
  TORQUE_LIMIT_COMMAND : Constant  Value=0
  UC_STATE : Constant  Value=UC_State.MC_Off
  VICOR_CURRENT : Constant  Value=0
  VSM_STATE : Constant  Value=MC_VSM_State.Start
  WATCHDOG : Constant  Value=0
  WHEEL_SPEED : Constant  Value=0
  Out Bus Element4 : Outport  PortName=Fault_Inputs  Element=Override_Ignition
  Out Bus Element1 : Outport  PortName=Fault_Inputs  Element=Ignition
  Out Bus Element2 : Outport  PortName=Fault_Inputs  Element=Override_ESTOP
  Out Bus Element3 : Outport  PortName=Fault_Inputs  Element=ESTOP
  Out Bus Element5 : Outport  PortName=Fault_Inputs  Element=Override_Brake
  Out Bus Element6 : Outport  PortName=Fault_Inputs  Element=Brake
  Out Bus Element7 : Outport  PortName=Fault_Inputs  Element=Override_Forward_EN
  Out Bus Element8 : Outport  PortName=Fault_Inputs  Element=Forward_EN
  Out Bus Element9 : Outport  PortName=Fault_Inputs  Element=Override_Start
  Out Bus Element10 : Outport  PortName=Fault_Inputs  Element=Start
  Out Bus Element11 : Outport  PortName=Fault_Inputs  Element=Override_Throttle
  Out Bus Element12 : Outport  PortName=Fault_Inputs  Element=Throttle
  Out Bus Element13 : Outport  PortName=Fault_Inputs  Element=Override_HIB_Comparison_Fault
  Out Bus Element14 : Outport  PortName=Fault_Inputs  Element=HIB_Comparison_Fault
  Out Bus Element15 : Outport  PortName=Fault_Inputs  Element=Override_Interlock
  Out Bus Element16 : Outport  PortName=Fault_Inputs  Element=Interlock
  Out Bus Element17 : Outport  PortName=Fault_Inputs  Element=Override_Inverter_Discharge_State
  Out Bus Element18 : Outport  PortName=Fault_Inputs  Element=Inverter_Discharge_State
  Out Bus Element19 : Outport  PortName=Fault_Inputs  Element=Override_LVSS_ON
  Out Bus Element20 : Outport  PortName=Fault_Inputs  Element=LVSS_ON
  Out Bus Element21 : Outport  PortName=Fault_Inputs  Element=Override_Contactor_Closed
  Out Bus Element22 : Outport  PortName=Fault_Inputs  Element=Contactor_Closed
  Out Bus Element23 : Outport  PortName=Fault_Inputs  Element=Override_Cell_Temps
  Out Bus Element24 : Outport  PortName=Fault_Inputs  Element=Cell_Temps
  Out Bus Element25 : Outport  PortName=Fault_Inputs  Element=Override_Cell_Voltages
  Out Bus Element26 : Outport  PortName=Fault_Inputs  Element=Cell_Voltages
  Out Bus Element27 : Outport  PortName=Fault_Inputs  Element=Override_Isolation_State
  Out Bus Element28 : Outport  PortName=Fault_Inputs  Element=Isolation_State
  Out Bus Element29 : Outport  PortName=Fault_Inputs  Element=Override_MC_Speed_Out
  Out Bus Element30 : Outport  PortName=Fault_Inputs  Element=MC_Speed_Out
  Out Bus Element31 : Outport  PortName=Fault_Inputs  Element=Override_Batt_Speed_Out
  Out Bus Element32 : Outport  PortName=Fault_Inputs  Element=Batt_Speed_Out
  Out Bus Element33 : Outport  PortName=Fault_Inputs  Element=Override_Temperatures
  Out Bus Element34 : Outport  PortName=Fault_Inputs  Element=Temperatures
  Out Bus Element35 : Outport  PortName=Fault_Inputs  Element=Override_MC_Flow_Rate
  Out Bus Element36 : Outport  PortName=Fault_Inputs  Element=MC_Flow_Rate
  Out Bus Element37 : Outport  PortName=Fault_Inputs  Element=Override_Batt_Flow_Rate
  Out Bus Element38 : Outport  PortName=Fault_Inputs  Element=Batt_Flow_Rate
  Out Bus Element39 : Outport  PortName=Fault_Inputs  Element=Override_HIB_ON
  Out Bus Element40 : Outport  PortName=Fault_Inputs  Element=HIB_ON
  Out Bus Element41 : Outport  PortName=Fault_Inputs  Element=Override_HUDL_ON
  Out Bus Element42 : Outport  PortName=Fault_Inputs  Element=HUDL_ON
  Out Bus Element43 : Outport  PortName=Fault_Inputs  Element=Override_TMS_ON
  Out Bus Element44 : Outport  PortName=Fault_Inputs  Element=TMS_ON
  Out Bus Element45 : Outport  PortName=Fault_Inputs  Element=Override_GUB_ON
  Out Bus Element46 : Outport  PortName=Fault_Inputs  Element=GUB_ON
  Out Bus Element47 : Outport  PortName=Fault_Inputs  Element=Override_Acc_ON
  Out Bus Element48 : Outport  PortName=Fault_Inputs  Element=Acc_ON
  Out Bus Element49 : Outport  PortName=Fault_Inputs  Element=Override_Batt_12V_ON
  Out Bus Element50 : Outport  PortName=Fault_Inputs  Element=Batt_12V_ON
  Out Bus Element51 : Outport  PortName=Fault_Inputs  Element=Override_Vicor_Current
  Out Bus Element52 : Outport  PortName=Fault_Inputs  Element=Vicor_Current
  Out Bus Element53 : Outport  PortName=Fault_Inputs  Element=Override_LVSS_Temps
  Out Bus Element54 : Outport  PortName=Fault_Inputs  Element=LVSS_Temps
  Out Bus Element55 : Outport  PortName=Fault_Inputs  Element=Override_LVSS_Currents
  Out Bus Element56 : Outport  PortName=Fault_Inputs  Element=LVSS_Currents
  Out Bus Element57 : Outport  PortName=Fault_Inputs  Element=Override_Heartbeats
  Out Bus Element58 : Outport  PortName=Fault_Inputs  Element=Heartbeats
  Out Bus Element59 : Outport  PortName=Fault_Inputs  Element=Override_MC_12V0
  Out Bus Element60 : Outport  PortName=Fault_Inputs  Element=MC_12V0
  Out Bus Element61 : Outport  PortName=Fault_Inputs  Element=Override_LVSS_EN
  Out Bus Element62 : Outport  PortName=Fault_Inputs  Element=LVSS_EN
  Out Bus Element63 : Outport  PortName=Fault_Inputs  Element=Override_nReset
  Out Bus Element64 : Outport  PortName=Fault_Inputs  Element=nReset
  Out Bus Element65 : Outport  PortName=Fault_Inputs  Element=Override_Self_Test
  Out Bus Element66 : Outport  PortName=Fault_Inputs  Element=Self_Test
  Out Bus Element67 : Outport  PortName=Fault_Inputs  Element=Override_Watchdog
  Out Bus Element68 : Outport  PortName=Fault_Inputs  Element=Watchdog
  Out Bus Element69 : Outport  PortName=Fault_Inputs  Element=Override_uC_State
  Out Bus Element70 : Outport  PortName=Fault_Inputs  Element=uC_State
  Out Bus Element71 : Outport  PortName=Fault_Inputs  Element=Override_VSM_State
  Out Bus Element72 : Outport  PortName=Fault_Inputs  Element=VSM_State
  Out Bus Element73 : Outport  PortName=Fault_Inputs  Element=Override_HB_Feedback
  Out Bus Element74 : Outport  PortName=Fault_Inputs  Element=HB_Feedback
  Out Bus Element75 : Outport  PortName=Fault_Inputs  Element=Override_HM_Fault
  Out Bus Element76 : Outport  PortName=Fault_Inputs  Element=HM_Fault
  Out Bus Element77 : Outport  PortName=Fault_Inputs  Element=Direction_Command
  Out Bus Element78 : Outport  PortName=Fault_Inputs  Element=Override_Direction_Command
  Out Bus Element79 : Outport  PortName=Fault_Inputs  Element=Rolling_Counter
  Out Bus Element80 : Outport  PortName=Fault_Inputs  Element=Override_Rolling_Counter
  Out Bus Element81 : Outport  PortName=Fault_Inputs  Element=Speed_Command
  Out Bus Element82 : Outport  PortName=Fault_Inputs  Element=Override_Speed_Command
  Out Bus Element83 : Outport  PortName=Fault_Inputs  Element=Speed_Mode_Enable
  Out Bus Element84 : Outport  PortName=Fault_Inputs  Element=Override_Speed_Mode_Enable
  Out Bus Element85 : Outport  PortName=Fault_Inputs  Element=Torque_Limit_Command
  Out Bus Element86 : Outport  PortName=Fault_Inputs  Element=Override_Torque_Limit_Command
  Out Bus Element87 : Outport  PortName=Fault_Inputs  Element=LS_Self_Test
  Out Bus Element88 : Outport  PortName=Fault_Inputs  Element=Override_LS_Self_Test
  Out Bus Element89 : Outport  PortName=Fault_Inputs  Element=MC_Self_Test
  Out Bus Element90 : Outport  PortName=Fault_Inputs  Element=Override_MC_Self_Test
  Out Bus Element91 : Outport  PortName=Fault_Inputs  Element=CAN_Self_Test
  Out Bus Element92 : Outport  PortName=Fault_Inputs  Element=Override_CAN_Self_Test
  Out Bus Element93 : Outport  PortName=Fault_Inputs  Element=LVSS_EN_Override
  Out Bus Element94 : Outport  PortName=Fault_Inputs  Element=Override_LVSS_EN_Override
  Out Bus Element95 : Outport  PortName=Fault_Inputs  Element=MC_EN_Override
  Out Bus Element96 : Outport  PortName=Fault_Inputs  Element=Override_MC_EN_Override
  Out Bus Element97 : Outport  PortName=Fault_Inputs  Element=CAN_Override
  Out Bus Element98 : Outport  PortName=Fault_Inputs  Element=Override_CAN_Override
  Out Bus Element99 : Outport  PortName=Fault_Inputs  Element=Wheel_Speed
  Out Bus Element100 : Outport  PortName=Fault_Inputs  Element=Override_Wheel_Speed
  wires:
  OVERRIDE_IGNITION/1 -> Data Type Conversion4/1
  Data Type Conversion4/1 -> Out Bus Element4/1
  Data Type Conversion1/1 -> Out Bus Element1/1
  IGNITION/1 -> Data Type Conversion1/1
  OVERRIDE_ESTOP/1 -> Data Type Conversion3/1
  Data Type Conversion2/1 -> Out Bus Element3/1
  ESTOP/1 -> Data Type Conversion2/1
  Data Type Conversion3/1 -> Out Bus Element2/1
  Data Type Conversion6/1 -> Out Bus Element5/1
  Data Type Conversion5/1 -> Out Bus Element6/1
  OVERRIDE_BRAKE/1 -> Data Type Conversion6/1
  BRAKE/1 -> Data Type Conversion5/1
  Data Type Conversion8/1 -> Out Bus Element7/1
  Data Type Conversion7/1 -> Out Bus Element8/1
  OVERRIDE_FORWARD_EN/1 -> Data Type Conversion8/1
  FORWARD_EN/1 -> Data Type Conversion7/1
  Data Type Conversion10/1 -> Out Bus Element9/1
  Data Type Conversion9/1 -> Out Bus Element10/1
  OVERRIDE_START/1 -> Data Type Conversion10/1
  START/1 -> Data Type Conversion9/1
  Data Type Conversion12/1 -> Out Bus Element11/1
  THROTTLE/1 -> Out Bus Element12/1
  OVERRIDE_THROTTLE/1 -> Data Type Conversion12/1
  HIB_COMPARISON/1 -> Data Type Conversion13/1
  Data Type Conversion14/1 -> Out Bus Element13/1
  OVERRIDE_HIB_COMPARISON/1 -> Data Type Conversion14/1
  Data Type Conversion13/1 -> Out Bus Element14/1
  INTERLOCK/1 -> Data Type Conversion15/1
  Data Type Conversion16/1 -> Out Bus Element15/1
  OVERRIDE_INTERLOCK/1 -> Data Type Conversion16/1
  Data Type Conversion15/1 -> Out Bus Element16/1
  Data Type Conversion18/1 -> Out Bus Element17/1
  OVERRIDE_INVERTER_DC_STATE/1 -> Data Type Conversion18/1
  LVSS_ON/1 -> Data Type Conversion19/1
  Data Type Conversion20/1 -> Out Bus Element19/1
  OVERRIDE_LVSS_ON/1 -> Data Type Conversion20/1
  Data Type Conversion19/1 -> Out Bus Element20/1
  BMS_CONTACTOR_CLOSED/1 -> Data Type Conversion21/1
  Data Type Conversion22/1 -> Out Bus Element21/1
  OVERRIDE_BMS_CONTACTOR_CLOSED/1 -> Data Type Conversion22/1
  Data Type Conversion21/1 -> Out Bus Element22/1
  CELL_TEMPS/1 -> Out Bus Element24/1
  Data Type Conversion23/1 -> Out Bus Element23/1
  OVERRIDE_CELL_TEMPS/1 -> Data Type Conversion23/1
  OVERRIDE_CELL_VOLTAGES/1 -> Data Type Conversion11/1
  Data Type Conversion11/1 -> Out Bus Element25/1
  CELL_VOLTAGES/1 -> Out Bus Element26/1
  OVERRIDE_ISOLATION_STATE/1 -> Data Type Conversion24/1
  Data Type Conversion24/1 -> Out Bus Element27/1
  ISOLATION_STATE/1 -> Out Bus Element28/1
  OVERRIDE_MC_SPEED_OUT/1 -> Data Type Conversion25/1
  Data Type Conversion25/1 -> Out Bus Element29/1
  MC_SPEED_OUT/1 -> Out Bus Element30/1
  BATT_SPEED_OUT/1 -> Out Bus Element32/1
  Data Type Conversion26/1 -> Out Bus Element31/1
  OVERRIDE_BATT_SPEED_OUT/1 -> Data Type Conversion26/1
  OVERRIDE_TEMPERATURES/1 -> Data Type Conversion27/1
  Data Type Conversion27/1 -> Out Bus Element33/1
  TEMPERATURES/1 -> Out Bus Element34/1
  MC_FLOW_RATE/1 -> Out Bus Element36/1
  Data Type Conversion28/1 -> Out Bus Element35/1
  OVERRIDE_MC_FLOW_RATE/1 -> Data Type Conversion28/1
  OVERRIDE_BATT_FLOW_RATE/1 -> Data Type Conversion29/1
  Data Type Conversion29/1 -> Out Bus Element37/1
  BATT_FLOW_RATE/1 -> Out Bus Element38/1
  Data Type Conversion30/1 -> Out Bus Element39/1
  OVERRIDE_HIB_ON/1 -> Data Type Conversion30/1
  HIB_ON/1 -> Data Type Conversion33/1
  Data Type Conversion31/1 -> Out Bus Element41/1
  OVERRIDE_HUDL_ON/1 -> Data Type Conversion31/1
  HUDL_ON/1 -> Data Type Conversion32/1
  Data Type Conversion32/1 -> Out Bus Element42/1
  Data Type Conversion33/1 -> Out Bus Element40/1
  Data Type Conversion35/1 -> Out Bus Element44/1
  TMS_ON/1 -> Data Type Conversion35/1
  Data Type Conversion34/1 -> Out Bus Element43/1
  OVERRIDE_TMS_ON/1 -> Data Type Conversion34/1
  Data Type Conversion37/1 -> Out Bus Element46/1
  GUB_ON/1 -> Data Type Conversion37/1
  Data Type Conversion36/1 -> Out Bus Element45/1
  OVERRIDE_GUB_ON/1 -> Data Type Conversion36/1
  Data Type Conversion39/1 -> Out Bus Element48/1
  ACC_ON/1 -> Data Type Conversion39/1
  Data Type Conversion38/1 -> Out Bus Element47/1
  OVERRIDE_ACC_ON/1 -> Data Type Conversion38/1
  Data Type Conversion41/1 -> Out Bus Element50/1
  BATT_12V_ON/1 -> Data Type Conversion41/1
  Data Type Conversion40/1 -> Out Bus Element49/1
  OVERRIDE_BATT_12V_ON/1 -> Data Type Conversion40/1
  VICOR_CURRENT/1 -> Out Bus Element52/1
  OVERRIDE_VICOR_CURRENT/1 -> Data Type Conversion42/1
  Data Type Conversion42/1 -> Out Bus Element51/1
  LVSS_TEMPS/1 -> Out Bus Element54/1
  OVERRIDE_LVSS_TEMPS/1 -> Data Type Conversion43/1
  Data Type Conversion43/1 -> Out Bus Element53/1
  LVSS_CURRENTS/1 -> Out Bus Element56/1
  OVERRIDE_LVSS_CURRENTS/1 -> Data Type Conversion44/1
  Data Type Conversion44/1 -> Out Bus Element55/1
  Data Type Conversion45/1 -> Out Bus Element57/1
  OVERRIDE_HEARTBEATS/1 -> Data Type Conversion45/1
  HEARTBEATS/1 -> Out Bus Element58/1
  Data Type Conversion46/1 -> Out Bus Element59/1
  MC_12V0/1 -> Data Type Conversion17/1
  OVERRIDE_MC_12V0/1 -> Data Type Conversion46/1
  Data Type Conversion17/1 -> Out Bus Element60/1
  OVERRIDE_LVSS_EN_UC/1 -> Data Type Conversion48/1
  Data Type Conversion48/1 -> Out Bus Element61/1
  LVSS_EN/1 -> Data Type Conversion47/1
  Data Type Conversion47/1 -> Out Bus Element62/1
  Data Type Conversion49/1 -> Out Bus Element64/1
  NRESET/1 -> Data Type Conversion49/1
  OVERRIDE_NRESET/1 -> Data Type Conversion50/1
  Data Type Conversion50/1 -> Out Bus Element63/1
  SELF_TEST/1 -> Out Bus Element66/1
  OVERRIDE_SELF_TEST/1 -> Data Type Conversion52/1
  Data Type Conversion52/1 -> Out Bus Element65/1
  Data Type Conversion51/1 -> Out Bus Element67/1
  OVERRIDE_WATCHDOG/1 -> Data Type Conversion51/1
  WATCHDOG/1 -> Data Type Conversion53/1
  Data Type Conversion53/1 -> Out Bus Element68/1
  Data Type Conversion54/1 -> Out Bus Element69/1
  OVERRIDE_UC_STATE/1 -> Data Type Conversion54/1
  Data Type Conversion55/1 -> Out Bus Element71/1
  OVERRIDE_VSM_STATE/1 -> Data Type Conversion55/1
  INVERTER_DC_STATE/1 -> Out Bus Element18/1
  VSM_STATE/1 -> Out Bus Element72/1
  UC_STATE/1 -> Out Bus Element70/1
  Data Type Conversion56/1 -> Out Bus Element73/1
  OVERRIDE_HB_FEEDBACK/1 -> Data Type Conversion56/1
  HB_FEEDBACK/1 -> Data Type Conversion57/1
  Data Type Conversion57/1 -> Out Bus Element74/1
  Data Type Conversion59/1 -> Out Bus Element76/1
  HM_FAULT/1 -> Data Type Conversion59/1
  OVERRIDE_HM_FAULT/1 -> Data Type Conversion58/1
  Data Type Conversion58/1 -> Out Bus Element75/1
  Data Type Conversion61/1 -> Out Bus Element83/1
  SPEED_MODE_ENABLE/1 -> Data Type Conversion61/1
  Data Type Conversion60/1 -> Out Bus Element77/1
  DIRECTION_COMMAND/1 -> Data Type Conversion60/1
  ROLLING_COUNTER/1 -> Data Type Conversion62/1
  Data Type Conversion62/1 -> Out Bus Element79/1
  Data Type Conversion63/1 -> Out Bus Element81/1
  TORQUE_LIMIT_COMMAND/1 -> Data Type Conversion64/1
  SPEED_COMMAND/1 -> Data Type Conversion63/1
  Data Type Conversion64/1 -> Out Bus Element85/1
  OVERRIDE_DIRECTION_COMMAND/1 -> Data Type Conversion65/1
  Data Type Conversion65/1 -> Out Bus Element78/1
  OVERRIDE_ROLLING_COUNTER/1 -> Data Type Conversion66/1
  Data Type Conversion66/1 -> Out Bus Element80/1
  OVERRIDE_SPEED_COMMAND/1 -> Data Type Conversion67/1
  Data Type Conversion67/1 -> Out Bus Element82/1
  OVERRIDE_SPEED_MODE_ENABLE/1 -> Data Type Conversion68/1
  Data Type Conversion68/1 -> Out Bus Element84/1
  OVERRIDE_TORQUE_LIMIT_COMMAND/1 -> Data Type Conversion69/1
  Data Type Conversion69/1 -> Out Bus Element86/1
  LS_SELF_TEST/1 -> Data Type Conversion70/1
  Data Type Conversion70/1 -> Out Bus Element87/1
  Data Type Conversion71/1 -> Out Bus Element88/1
  OVERRIDE_LS_SELF_TEST/1 -> Data Type Conversion71/1
  OVERRIDE_MC_SELF_TEST/1 -> Data Type Conversion73/1
  Data Type Conversion73/1 -> Out Bus Element90/1
  Data Type Conversion72/1 -> Out Bus Element89/1
  MC_SELF_TEST/1 -> Data Type Conversion72/1
  CAN_SELF_TEST/1 -> Data Type Conversion74/1
  Data Type Conversion74/1 -> Out Bus Element91/1
  Data Type Conversion75/1 -> Out Bus Element92/1
  OVERRIDE_CAN_SELF_TEST/1 -> Data Type Conversion75/1
  Data Type Conversion76/1 -> Out Bus Element93/1
  LVSS_EN_OVERRIDE/1 -> Data Type Conversion76/1
  Data Type Conversion77/1 -> Out Bus Element94/1
  OVERRIDE_LVSS_EN_OVERRIDE/1 -> Data Type Conversion77/1
  Data Type Conversion78/1 -> Out Bus Element95/1
  MC_EN_OVERRIDE/1 -> Data Type Conversion78/1
  Data Type Conversion79/1 -> Out Bus Element96/1
  OVERRIDE_MC_EN_OVERRIDE/1 -> Data Type Conversion79/1
  CAN_OVERRIDE/1 -> Data Type Conversion80/1
  Data Type Conversion81/1 -> Out Bus Element98/1
  OVERRIDE_CAN_OVERRIDE/1 -> Data Type Conversion81/1
  Data Type Conversion80/1 -> Out Bus Element97/1
  Data Type Conversion83/1 -> Out Bus Element100/1
  WHEEL_SPEED/1 -> Out Bus Element99/1
  OVERRIDE_WHEEL_SPEED/1 -> Data Type Conversion83/1

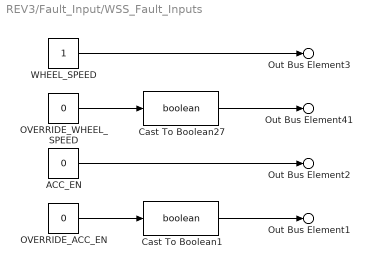
== system REV3/Fault_Input/WSS_Fault_Inputs ==
  ACC_EN : Constant  Value=0
  Cast To Boolean1 : DataTypeConversion  OutDataTypeStr=boolean  SaturateOnIntegerOverflow=off  RndMeth=Floor
  Cast To Boolean27 : DataTypeConversion  OutDataTypeStr=boolean  SaturateOnIntegerOverflow=off  RndMeth=Floor
  OVERRIDE_ACC_EN : Constant  Value=0
  OVERRIDE_WHEEL_SPEED : Constant  Value=0
  WHEEL_SPEED : Constant
  Out Bus Element41 : Outport  PortName=Fault_Inputs  Element=Override_Wheel_Speed
  Out Bus Element1 : Outport  PortName=Fault_Inputs  Element=Override_Acc_EN
  Out Bus Element2 : Outport  PortName=Fault_Inputs  Element=Acc_EN
  Out Bus Element3 : Outport  PortName=Fault_Inputs  Element=Wheel_Speed
  wires:
  OVERRIDE_WHEEL_SPEED/1 -> Cast To Boolean27/1
  Cast To Boolean27/1 -> Out Bus Element41/1
  ACC_EN/1 -> Out Bus Element2/1
  OVERRIDE_ACC_EN/1 -> Cast To Boolean1/1
  Cast To Boolean1/1 -> Out Bus Element1/1
  WHEEL_SPEED/1 -> Out Bus Element3/1

== system REV3/Plant_Model/Bike_Orientation ==

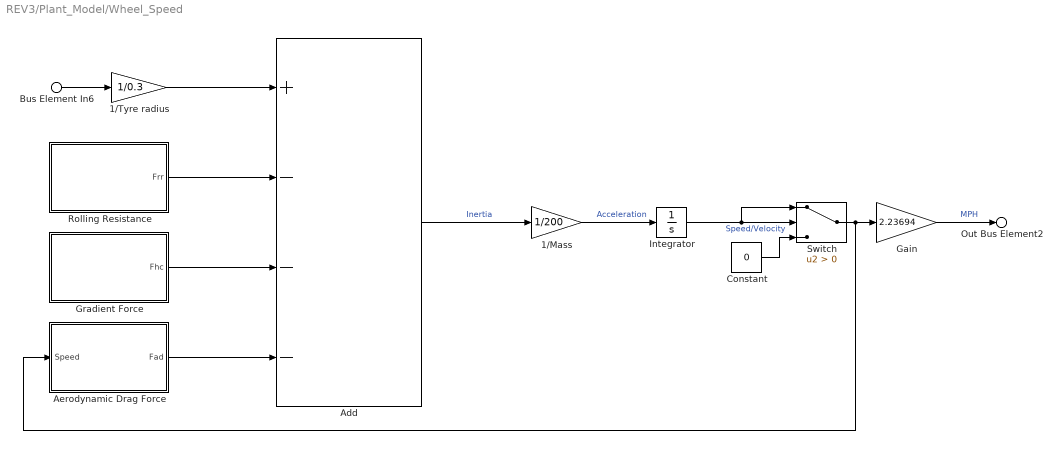
== system REV3/Plant_Model/Wheel_Speed ==
  Bus Element In6 : Inport  PortName=Motor_Outputs  Element=Torque
  1/Mass : Gain  Gain=1/200
  1/Tyre radius : Gain  Gain=1/0.3
  Add : Sum  Inputs=+---
  Aerodynamic Drag Force : Subsystem
  Constant : Constant  Value=0
  Gain : Gain  Gain=2.23694
  Gradient Force : Subsystem
  Integrator : Integrator
  Rolling Resistance : Subsystem
  Switch : Switch  Criteria=u2 > Threshold  SaturateOnIntegerOverflow=off  InputSameDT=off
  Out Bus Element2 : Outport  PortName=Plant_Model_Outputs  Element=WSS_Wheel_Speed
  wires:
  Aerodynamic Drag Force/1(Fad) -> Add/4
  Gain/1 -> Out Bus Element2/1  "MPH"
  Add/1 -> 1/Mass/1  "Inertia"
  Switch/1 -> Aerodynamic Drag Force/1(Speed), Gain/1
  Integrator/1 -> Switch/1, Switch/2  "Speed/Velocity"
  Gradient Force/1(Fhc) -> Add/3
  Rolling Resistance/1(Frr) -> Add/2
  1/Mass/1 -> Integrator/1  "Acceleration"
  Constant/1 -> Switch/3
  1/Tyre radius/1 -> Add/1
  Bus Element In6/1 -> 1/Tyre radius/1
